simulink model "ensaio"  (Simulink 8.5)
settings: Solver=ode4  SolverMode=SingleTasking  StartTime=0.0  StopTime=80  FixedStep=0.001  RelTol=1e-3
undefined symbols (not defined in the file): Kd_pid1, Kd_pid2, Kd_pid3, Kd_pid4, Kd_pid5, Ki_pid1, Ki_pid2, Ki_pid3, Ki_pid4, Ki_pid5, Kp_pid1, Kp_pid2, Kp_pid3, Kp_pid4, Kp_pid5, N_pid1, N_pid2, N_pid3, N_pid4, N_pid5, sigbuilder_block
libraries: simulink_extras x2, simulink x1
settings Model: Creator=colom  LastModifiedBy=colom  SimulationMode=accelerator  CovMetricSettings=dwe  CovHtmlReporting=off  covSaveCumulativeToWorkspaceVar=off  CovSaveSingleToWorkspaceVar=off  CovExternalEMLEnable=on
settings SolverCC: AutoInsertRateTranBlk=on
settings DataIOCC: LimitDataPoints=off  SaveFormat=Dataset  SignalLoggingSaveFormat=Dataset  ReturnWorkspaceOutputs=on
settings OptimizationCC: ExpressionDepthLimit=128
settings DebuggingCC: UnderspecifiedInitializationDetection=Simplified  MergeDetectMultiDrivingBlocksExec=error  FcnCallInpInsideContextMsg=EnableAllAsError  UnconnectedInputMsg=none  UnconnectedOutputMsg=none  UnconnectedLineMsg=none  StateNameClashWarn=none  SFUnexpectedBacktrackingDiag=error  SFNoUnconditionalDefaultTransitionDiag=error
settings HardwareCC: ProdBitPerPointer=64  ProdLargestAtomicFloat=Float  ProdIntDivRoundTo=Zero  ProdEndianess=LittleEndian  ProdHWDeviceType=Specified
settings ModelReferenceCC: PropagateSignalLabelsOutOfModel=on
settings SFSimCC: SimUseLocalCustomCode=on
settings RTWCC: RTWUseLocalCustomCode=on
settings GRTTargetCC: TargetLangStandard=C99 (ISO)  CombineOutputUpdateFcns=on  GRTInterface=off

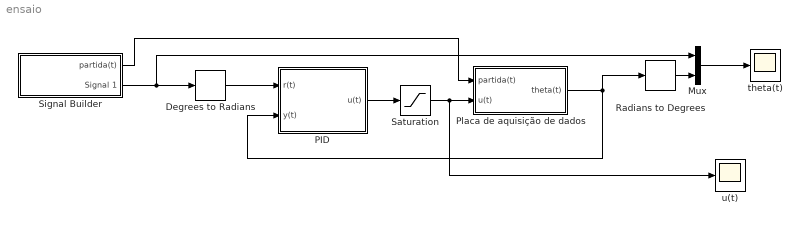
== system ensaio ==
  Degrees to Radians : simulink_extras/Transformations/Degrees to Radians
  Mux : Mux  Inputs=2
  PID : Subsystem
  Placa de aquisição de dados : Subsystem
  Radians to Degrees : simulink_extras/Transformations/Radians to Degrees
  Saturation : Saturate  UpperLimit=100  LowerLimit=0
  Signal Builder : Subsystem  Tag=STV Subsys  LoadFcn=sigbuilder_block('load');  StartFcn=sigbuilder_block('start');  StopFcn=sigbuilder_block('stop');  ClipboardFcn=sigbuilder_block('clipboard');  mask(Sigbuilder block){}
      mask help: Simulink:masks:SigbuilderBlock_MD
      mask init:
      | if ~strcmp(get_param(bdroot(gcbh),'SimulationStatus'),'stopped') tuvar = sigbuilder_block('maskInit'); end
      settings: CopyFcn=sigbuilder_block('copy');  DeleteFcn=sigbuilder_block('delete');  ModelCloseFcn=sigbuilder_block('modelClose');  PreSaveFcn=sigbuilder_block('preSave');  PauseFcn=sigbuilder_block('pause');  ContinueFcn=sigbuilder_block('continue');  NameChangeFcn=sigbuilder_block('namechange');  OpenFcn=sigbuilder_block('open',[302.25 165 1093.5 399.75 ]);  CloseFcn=sigbuilder_block('close');
      mask Display: plot(0, 0, 100, 100,[2, 2, 32, 32, 2], [68, 8, 8, 68, 68],[32, 2], [38, 38], [32, 19, 2],[53, 60, 44], [32, 17, 17, 2],[16, 16, 31, 31]);txt = getActiveGroup(gcbh);text(2, 100, txt,'verticalAlignment', 'top');
  theta(t) : Scope
      settings: TimeRange=80  YMin=0  YMax=190
  u(t) : Scope
      settings: TimeRange=30  YMin=0  YMax=100
  wires:
  Signal Builder/1(partida(t)) -> Placa de aquisição de dados/1(partida(t))
  Degrees to Radians/1 -> PID/1(r(t))
  Saturation/1 -> Placa de aquisição de dados/2(u(t)), u(t)/1
  PID/1(u(t)) -> Saturation/1
  Signal Builder/2(Signal 1) -> Mux/1, Degrees to Radians/1
  Placa de aquisição de dados/1(theta(t)) -> PID/2(y(t)), Radians to Degrees/1
  Mux/1 -> theta(t)/1
  Radians to Degrees/1 -> Mux/2

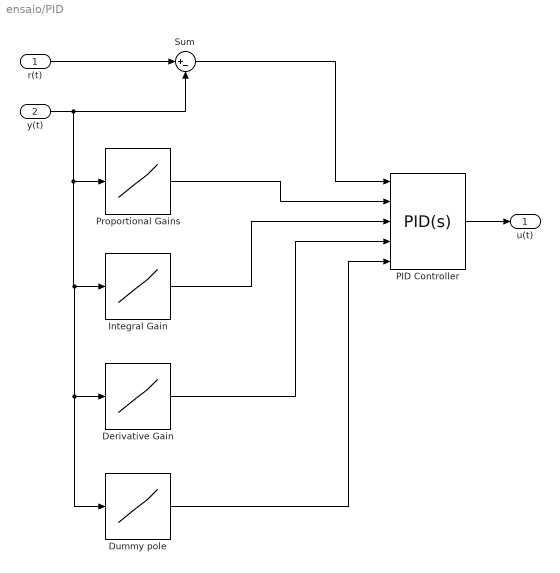
== system ensaio/PID ==
  r(t) : Inport
  y(t) : Inport  Port=2
  Derivative Gain : Lookup_n-D  NumberOfTableDimensions=1  BreakpointsForDimension1=deg2rad([15 37.5 55 70 85])  BreakpointsForDimension2=[-5:5]  BreakpointsForDimension3=[-5:5]  BreakpointsForDimension4=[-5:5]  Table=[Kd_pid1 Kd_pid2 Kd_pid3 Kd_pid4 Kd_pid5]  InternalRulePriority=Speed  RndMeth=Simplest  InputSameDT=on
  Dummy pole : Lookup_n-D  NumberOfTableDimensions=1  BreakpointsForDimension1=deg2rad([15 37.5 55 70 85])  BreakpointsForDimension2=[-5:5]  BreakpointsForDimension3=[-5:5]  BreakpointsForDimension4=[-5:5]  Table=[N_pid1 N_pid2 N_pid3 N_pid4 N_pid5]  InternalRulePriority=Speed  RndMeth=Simplest  InputSameDT=on
  Integral Gain : Lookup_n-D  NumberOfTableDimensions=1  BreakpointsForDimension1=deg2rad([15 37.5 55 70 85])  BreakpointsForDimension2=[-5:5]  BreakpointsForDimension3=[-5:5]  BreakpointsForDimension4=[-5:5]  Table=[Ki_pid1 Ki_pid2 Ki_pid3 Ki_pid4 Ki_pid5]  InternalRulePriority=Speed  RndMeth=Simplest  InputSameDT=on
  PID Controller : simulink/Continuous/PID Controller  Controller=PID  TimeDomain=Continuous-time  SampleTime=-1  IntegratorMethod=Forward Euler  FilterMethod=Forward Euler  Form=Parallel  UseFilter=on  ControllerParametersSource=external  P=1  I=1  D=0  N=100  InitialConditionSource=internal  InitialConditionForIntegrator=0  InitialConditionForFilter=0  ExternalReset=none  LimitOutput=off  UpperSaturationLimit=inf  LowerSaturationLimit=-inf  LinearizeAsGain=on  AntiWindupMode=none  Kb=1  TrackingMode=off  Kt=1  PParamMin=[]  PParamMax=[]  IParamMin=[]  IParamMax=[]  DParamMin=[]  DParamMax=[]  NParamMin=[]  NParamMax=[]  KbParamMin=[]  KbParamMax=[]  KtParamMin=[]  KtParamMax=[]  POutMin=[]  POutMax=[]  IOutMin=[]  IOutMax=[]  DOutMin=[]  DOutMax=[]  NOutMin=[]  NOutMax=[]  KbOutMin=[]  KbOutMax=[]  KtOutMin=[]  KtOutMax=[]  IntegratorOutMin=[]  IntegratorOutMax=[]  FilterOutMin=[]  FilterOutMax=[]  SumOutMin=[]  SumOutMax=[]  SumI1OutMin=[]  SumI1OutMax=[]  SumI2OutMin=[]  SumI2OutMax=[]  SumI3OutMin=[]  SumI3OutMax=[]  SumDOutMin=[]  SumDOutMax=[]  SaturationOutMin=[]  SaturationOutMax=[]  IntegratorContinuousStateAttributes=''  IntegratorStateMustResolveToSignalObject=off  IntegratorRTWStateStorageClass=Auto  FilterContinuousStateAttributes=''  FilterStateMustResolveToSignalObject=off  FilterRTWStateStorageClass=Auto  DifferentiatorICPrevScaledInput=0  DifferentiatorOutMin=[]  DifferentiatorOutMax=[]
  Proportional Gains : Lookup_n-D  NumberOfTableDimensions=1  BreakpointsForDimension1=deg2rad([15 37.5 55 70 85])  BreakpointsForDimension2=[-5:5]  BreakpointsForDimension3=[-5:5]  BreakpointsForDimension4=[-5:5]  Table=[Kp_pid1 Kp_pid2 Kp_pid3 Kp_pid4 Kp_pid5]  InternalRulePriority=Speed  RndMeth=Simplest  InputSameDT=on
  Sum : Sum  Inputs=|+-
  u(t) : Outport
  wires:
  y(t)/1 -> Dummy pole/1, Derivative Gain/1, Integral Gain/1, Proportional Gains/1, Sum/2
  r(t)/1 -> Sum/1
  PID Controller/1 -> u(t)/1
  Dummy pole/1 -> PID Controller/5
  Proportional Gains/1 -> PID Controller/2
  Sum/1 -> PID Controller/1
  Integral Gain/1 -> PID Controller/3
  Derivative Gain/1 -> PID Controller/4

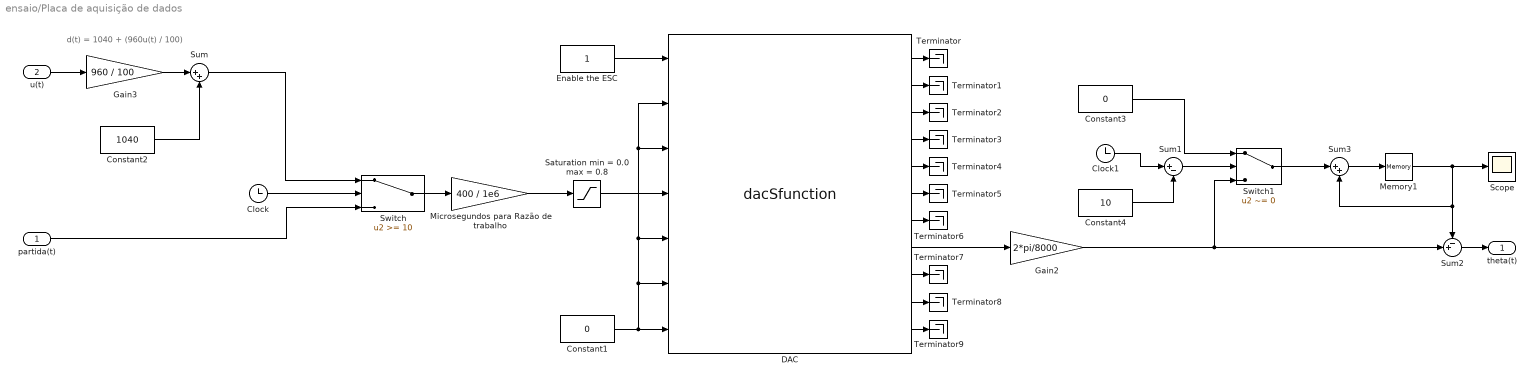
== system ensaio/Placa de aquisição de dados ==
  note: d(t) = 1040 + (960u(t) / 100)
  partida(t) : Inport
  u(t) : Inport  Port=2
  Clock : Clock
  Clock1 : Clock
  Constant1 : Constant  Value=0
  Constant2 : Constant  Value=1040
  Constant3 : Constant  Value=0
  Constant4 : Constant  Value=10
  DAC : S-Function  FunctionName=dacSfunction  Parameters=serialPort,sampleTime,gpioOutCh1FinalState,gpioOutCh2FinalState,gpioOutCh3FinalState,pwmFrequency,pwmCh1FinalDuty,pwmCh2FinalDuty,pwmCh3FinalDuty,pwmCh4FinalDuty,enc1Mode,enc1ResetCount,enc1Direction,enc1Quadrature,enc1Filter,enc2Mode,enc2ResetCount,enc2Direction,enc2Quadrature,enc2Filter,enc3Mode,enc3ResetCount,enc3Direction,enc3Quadrature,enc3Filter  mask{serialPort='COM9', sampleTime=10, gpioOutCh1FinalState=Low, gpioOutCh2FinalState=Low, gpioOutCh3FinalState=Low, pwmFrequency=400, pwmCh1FinalDuty=0, pwmCh2FinalDuty=0, pwmCh3FinalDuty=0, pwmCh4FinalDuty=0, enc1Mode=Counter, enc1Direction=Counter Clock Wise is positive, enc1Quadrature=High resolution, enc1Filter=15, enc1ResetCount=on, enc2Mode=Counter, enc2Direction=Counter Clock Wise is positive, enc2Quadrature=High resolution, enc2Filter=15, enc2ResetCount=off, enc3Mode=Counter, enc3Direction=Clock Wise is positive, enc3Quadrature=High resolution, enc3Filter=15, enc3ResetCount=off}
      mask prompts: serialPort "Serial port"; sampleTime "Sample time (ms)"; gpioOutCh1FinalState "Final state"; gpioOutCh2FinalState "Final state"; gpioOutCh3FinalState "Final state"; pwmFrequency "Frequency (Hz)"; pwmCh1FinalDuty "Final duty"; pwmCh2FinalDuty "Final duty"; pwmCh3FinalDuty "Final duty"; pwmCh4FinalDuty "Final duty"; enc1Mode "Mode"; enc1Direction "Direction"; enc1Quadrature "Resolution"; enc1Filter "Filter"; enc1ResetCount "Reset count"; enc2Mode "Mode"; enc2Direction "Direction"; enc2Quadrature "Resolution"; enc2Filter "Filter"; enc2ResetCount "Reset count"; enc3Mode "Mode"; enc3Direction "Direction"; enc3Quadrature "Resolution"; enc3Filter "Filter"; enc3ResetCount "Reset count"
      mask init:
      | % The first list item is initiated with 1 and not 0
      mask TypeOptions gpioOutCh1FinalState: Low | High
      mask TypeOptions gpioOutCh2FinalState: Low | High
      mask TypeOptions gpioOutCh3FinalState: Low | High
      mask TypeOptions enc1Mode: Counter | Time measurement
      mask TypeOptions enc1Direction: Counter Clock Wise is positive | Clock Wise is positive
      mask TypeOptions enc1Quadrature: Low resolution | High resolution
      mask TypeOptions enc2Mode: Counter | Time measurement
      mask TypeOptions enc2Direction: Counter Clock Wise is positive | Clock Wise is positive
      mask TypeOptions enc2Quadrature: Low resolution | High resolution
      mask TypeOptions enc3Mode: Counter | Time measurement
      mask TypeOptions enc3Direction: Counter Clock Wise is positive | Clock Wise is positive
      mask TypeOptions enc3Quadrature: Low resolution | High resolution
      mask DialogControl DescTextVar Prompt: %<MaskDescription> OpenDAC configuration
      mask Display:
      | % Give names to the input ports
      | port_label('input', 1, 'Digital Out CH1 (PC15)');
      | port_label('input', 2, 'Digital Out CH2 (PC14)');
      | port_label('input', 3, 'Digital Out CH3 (PC13)');
      | port_label('input', 4, 'PWM CH1 (PB6)');
      | port_label('input', 5, 'PWM CH2 (PB7)');
      | port_label('input', 6, 'PWM CH3 (PB8)');
      | port_label('input', 7, 'PWM CH4 (PB9)');
      | 
      | % Give names to the output ports
      | port_label('output', 1, 'Digital In CH1 (PB12)');
      | port_label('output', 2, 'Digital In CH2 (PB13)');
      | port_label('output', 3, 'Digital In CH3 (PB14)');
      | port_label('output', 4, 'Analog In CH1 (PA0)');
      | port_label('output', 5, 'Analog In CH2 (PA1)');
      | port_label('output', 6, 'Analog In CH3 (PA4)');
      | port_label('output', 7, 'Analog In CH4 (PB0)');
      | port_label('output', 8, 'Encoder 1 (PA8/PA9)');
      | port_label('output', 9, 'Encoder 2 (PA15/PB3)');
      | port_label('output', 10, 'Encoder 3 (PB4/PB5)');
      | port_label('output', 11, 'Real Time Clock');
  Enable the ESC : Constant
  Gain2 : Gain  Gain=2*pi/8000
  Gain3 : Gain  Gain=960 / 100
  Memory1 : Memory
  Microsegundos para Razão de trabalho : Gain  Gain=400 / 1e6
  Saturation min = 0.0 max = 0.8 : Saturate  UpperLimit=0.8  LowerLimit=0.0
  Scope : Scope
      settings: TimeRange=20  YMin=0  YMax=3  SaveName=ScopeData2
  Sum : Sum  Inputs=|++
  Sum1 : Sum  Inputs=|+-
  Sum2 : Sum  Inputs=-+|
  Sum3 : Sum  Inputs=|++
  Switch : Switch  Threshold=10
  Switch1 : Switch  Criteria=u2 ~= 0
  Terminator{,1..9} (10 alike) : Terminator
  theta(t) : Outport
  wires:
  DAC/8 -> Gain2/1
  Constant1/1 -> DAC/3, DAC/2, DAC/5, DAC/6, DAC/7
  Enable the ESC/1 -> DAC/1
  Gain2/1 -> Switch1/3, Sum2/2
  Gain3/1 -> Sum/1
  Constant2/1 -> Sum/2
  DAC/2 -> Terminator1/1
  DAC/1 -> Terminator/1
  DAC/3 -> Terminator2/1
  DAC/4 -> Terminator3/1
  DAC/5 -> Terminator4/1
  DAC/6 -> Terminator5/1
  DAC/7 -> Terminator6/1
  DAC/9 -> Terminator7/1
  DAC/10 -> Terminator8/1
  DAC/11 -> Terminator9/1
  Saturation min = 0.0 max = 0.8/1 -> DAC/4
  u(t)/1 -> Gain3/1
  Microsegundos para Razão de trabalho/1 -> Saturation min = 0.0 max = 0.8/1
  Switch/1 -> Microsegundos para Razão de trabalho/1
  Clock/1 -> Switch/2
  Sum/1 -> Switch/1
  partida(t)/1 -> Switch/3
  Sum2/1 -> theta(t)/1
  Memory1/1 -> Sum3/2, Sum2/1, Scope/1
  Switch1/1 -> Sum3/1
  Sum3/1 -> Memory1/1
  Constant3/1 -> Switch1/1
  Clock1/1 -> Sum1/1
  Constant4/1 -> Sum1/2
  Sum1/1 -> Switch1/2

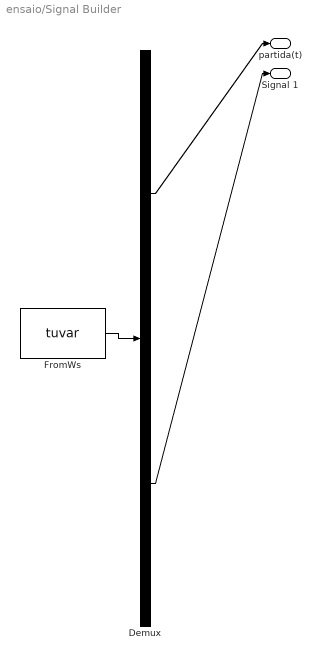
== system ensaio/Signal Builder ==
  Demux : Demux  Tag=STV Demux  Outputs=2
  FromWs : FromWorkspace  Tag=STV FromWs  VariableName=tuvar  SampleTime=0  SigBuilderData=DataTag0  VnvData=DataTag1
      SigBuilderData=|
      | common.afterFinalStr = 'Extrapolate'
      | common.sampleTime = 0
      | dataSet.timeRange = [0 80]
      | dataSet.name = 'Group 1'
      | sbobj.Groups.Name = 'Group 1'
      | sbobj.Groups.Signals(1).Name = 'partida(t)'
      | sbobj.Groups.Signals(1).XData = [0 0.5 0.5 2.5 2.5 6.5 6.5 10 10 15 16 17 18 19 80]
      | sbobj.Groups.Signals(1).YData = [0 0 2000 2000 2 0 1040 1040 4 0 0 0 0 0 0]
      | sbobj.Groups.Signals(2).Name = 'Signal 1'
      | sbobj.Groups.Signals(2).XData = [0 11 15 20 23 28 31 36 39 44 44 47 52 52 72 73 74 75 76 77 78 79 80]
      | sbobj.Groups.Signals(2).YData = [0 0 20 20 40 40 60 60 75 75 85 85 85 75 0 0 0 0 0 0 0 0 0]
      | sbobj.Groups.TimeRange = [0 80]
  partida(t) : Outport  Tag=STV Outport
  Signal 1 : Outport  Tag=STV Outport  Port=2
  wires:
  FromWs/1 -> Demux/1
  Demux/1 -> partida(t)/1
  Demux/2 -> Signal 1/1
